simulink model "afti16sim"  (Simulink 8.8)
settings: Solver=ode45  StartTime=0.0  StopTime=Tstop  RelTol=1e-3
values from neighbouring files (symbols this model uses):
  A = [-.0151 -60.5651 0 -32.174 ... (first row only)    [afti16.m]    (also in bmdp02.m = [0.7326   -0.0861; example4.m = [1 -1 0; regulator.m = [0 0; sphericle.m = [0 0 1 0;0 0 0 1 ;-66.2175 66.2175 -0.15 0 ;0 0 0 0])
  B = [-2.516 -13.136 ... (first row only)    [afti16.m]    (also in bmdp02.m = [0.0609;0.0064]; example4.m = [-1 1; regulator.m = [1;0]; sphericle.m = [0 0 0 1]')
  C = [0 1 0 0 ... (first row only)    [afti16.m]    (also in bmdp02.m = lincon(model,'reg',cost,interval,limits); example4.m = lincon(model,'reg',cost,interval,limits); mimo.m = lincon(model,'track',cost,interval,limits); regsiso.m = model.C)
  Cf16 = lincon(model,'track',cost,interval,limits)    [afti16.m]
  D = [0 0 ... (first row only)    [afti16.m]    (also in bmdp02.m = zeros(size(B)); example4.m = zeros(2,2); regulator.m = 0; sphericle.m = 0)
  sp = [0 20]    [afti16.m]    (also in mimo.m = [0.63 0.79]')
  x0 = zeros(4,1)    [afti16.m]    (also in bmdp02.m = [1 1]'; dcmotor.m; doubleint.m = [10,-.3]'; doubleintexp.m = [10,-.3]')
libraries: hyblib x1
settings Model: SuppressorTable=22 serialization::archive 11 0 3 0 0 0 0 0  Creator=bemporad  LastModifiedBy=bemporad  ExtModeTrigMode=oneshot  ExtModeArmWhenConnect=off
settings DataIOCC: LimitDataPoints=off  SignalLoggingName=sigsOut
settings OptimizationCC: BooleanDataType=off  LifeSpan=auto
settings DebuggingCC: SaveWithParameterizedLinksMsg=none  SignalResolutionControl=TryResolveAllWithWarning  MultiTaskDSMMsg=warning  MultiTaskCondExecSysMsg=none  IntegerOverflowMsg=none  FcnCallInpInsideContextMsg=error  StateNameClashWarn=none  SFUnexpectedBacktrackingDiag=error  SFNoUnconditionalDefaultTransitionDiag=error  SFExecutionAtInitializationDiag=warning
settings HardwareCC: TargetUnknown=on
settings GRTTargetCC: GeneratePreprocessorConditionals=Use local settings

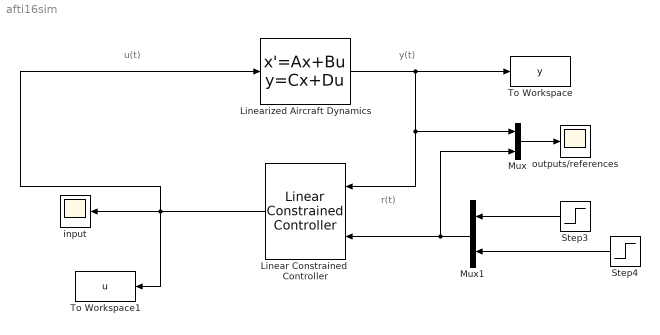
== system afti16sim ==
  note: u(t)
  note: y(t)
  note: r(t)
  Linear Constrained  Controller : hyblib/Linear Constrained  Controller  C=Cf16  xhat0=[]  u1=[]
  Linearized Aircraft Dynamics : StateSpace  A=A  B=B  C=C  D=D  X0=x0
  Mux : Mux  Inputs=2
  Mux1 : Mux  Inputs=2
  Step3 : Step  Time=0  After=sp(1)  SampleTime=0
  Step4 : Step  Time=0  After=sp(2)  SampleTime=0
  To Workspace : ToWorkspace  VariableName=y  SampleTime=-1
  To Workspace1 : ToWorkspace  VariableName=u  SampleTime=-1
  input : Scope
  outputs/references : Scope
  wires:
  Linearized Aircraft Dynamics/1 -> To Workspace/1, Linear Constrained  Controller/1, Mux/1
  Mux/1 -> outputs/references/1
  Linear Constrained  Controller/1 -> To Workspace1/1, input/1, Linearized Aircraft Dynamics/1
  Step3/1 -> Mux1/1
  Step4/1 -> Mux1/2
  Mux1/1 -> Mux/2, Linear Constrained  Controller/2
